simulink model "linear_all"  (R2016b)
settings: Solver=VariableStepAuto  StartTime=0.0  StopTime=100  RelTol=1e-3
values from neighbouring files (symbols this model uses):
  K_ball = get(P_ball, 'D')    [calculate_cascade.m]
  K_beam = [-8.20687974687 -1.57558991566]    [beam_linearization_controller.mat]    (also in calculate_cascade.m = get(P_beam, 'D'))
libraries: cstblocks x2
settings Model: Creator=piotr  LastModifiedBy=piotr

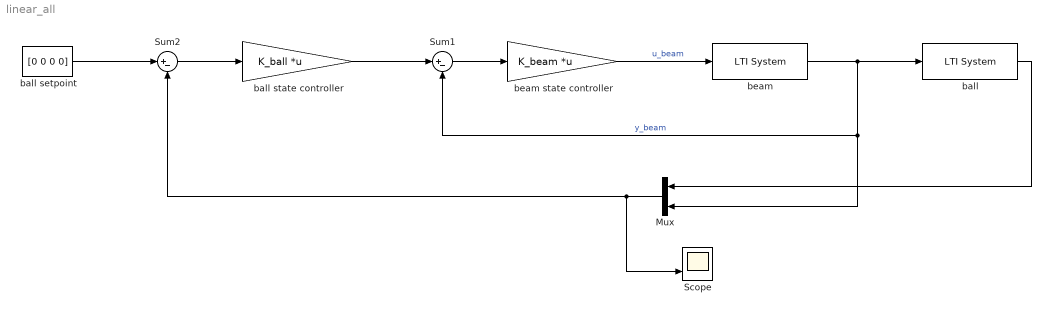
== system linear_all ==
  Mux : Mux  Inputs=2
  Scope : Scope  NumInputPorts=2
  Sum1 : Sum  Inputs=|+-
  Sum2 : Sum  Inputs=|+-
  ball : cstblocks/LTI System  sys=ball_SS  IC=[0.2 0]
  ball setpoint : Constant  Value=[0 0 0 0]
  ball state controller : Gain  Gain=K_ball  Multiplication=Matrix(K*u) (u vector)
  beam : cstblocks/LTI System  sys=beam_SS  IC=[-0.3 0]
  beam state controller : Gain  Gain=K_beam  Multiplication=Matrix(K*u) (u vector)
  wires:
  beam state controller/1 -> beam/1  "u_beam"
  beam/1 -> Mux/2, Sum1/2, ball/1  "y_beam"
  Sum1/1 -> beam state controller/1
  ball setpoint/1 -> Sum2/1
  Sum2/1 -> ball state controller/1
  ball state controller/1 -> Sum1/1
  ball/1 -> Mux/1
  Mux/1 -> Scope/2, Sum2/2
